simulink model "ConSys_A1"  (Simulink 8.3)
settings: Solver=ode3  StartTime=0.0  StopTime=Time(end)  FixedStep=Ts  RelTol=1e-3
values from neighbouring files (symbols this model uses):
  d = r*h    (= 1.6)    [StartUp_A1.m]
  d0 = d*h    (= 0.0032)    [StartUp_A1.m]
  h = 0.002    [StartUp_A1.m]
  Ka = diag([ 3  20  20  150  355  520])    [StartUp_A1.m]
  Kd = diag([ 3   5  25  100   15 1050])    [StartUp_A1.m]
  Ki = diag([35 555 810 7410 1850 5815])    [StartUp_A1.m]
  Kp = diag([55 180 350 1960  680 4450])    [StartUp_A1.m]
  r = 800    [StartUp_A1.m]
  TD = ss(Atd,Btd,Ctd,Dtd,Ts)    [StartUp_A1.m]
  Ts = 1/200    (= 0.005)    [StartUp_A1.m]
undefined symbols (not defined in the file or in its folder): DiscIntNeverNeededParam
undefined symbols (not defined in the file): ADAMS_cwd, ADAMS_exec, ADAMS_host, ADAMS_init, ADAMS_inputs, ADAMS_outputs, ADAMS_prefix, ADAMS_static, ADAMS_sysdir
libraries: cstblocks x6
(part 5 of 9)

== matlab function A2/MATLAB Function 2 ==
  data: q input double; V2 output double; dq input double
function V2 = V2(q,dq)
%#codegen
Th1=q(1,1); Th2=q(2,1); Th3=q(3,1); Th4=q(4,1); Th5=q(5,1); Th6=q(6,1);
dTh1=dq(1); dTh2=dq(2); dTh3=dq(3); dTh4=dq(4); dTh5=dq(5); dTh6=dq(6);
%---------------------------
V211=(0.34701*cos(Th2) - 0.50841*sin(2.0*Th2) - 0.006265*cos(2.0*Th2 + 2.0*Th3) - 0.04536*cos(2.0*Th2) + 1.3719*sin(2.0*Th2 + 2.0*Th3) - 0.017028*sin(Th2) - 0.096468*cos(Th2)^2 + (0.55399*sin(Th2 + Th3) + 2.34*cos(Th2) + 1.651*cos(Th2)*sin(Th3) + 1.651*cos(Th3)*sin(Th2))*(0.08523*cos(Th2 + Th3) - 0.36*sin(Th2) + 0.254*cos(Th2)*cos(Th3) - 0.254*sin(Th2)*sin(Th3) + 0.07) - 0.5*(cos(Th6)*(sin(Th2 + Th3)*sin(Th5) - 1.0*cos(Th2 + Th3)*cos(Th4)*cos(Th5)) + cos(Th2 + Th3)*sin(Th4)*sin(Th6))*(0.001043*cos(Th6)*(cos(Th2 + Th3)*sin(Th5) + sin(Th2 + Th3)*cos(Th4)*cos(Th5)) - 4.0e-6*cos(Th2 + Th3)*cos(Th5) + 4.0e-6*sin(Th2 + Th3)*cos(Th4)*sin(Th5) - 0.001043*sin(Th2 + Th3)*sin(Th4)*sin(Th6)) - 0.004943*cos(Th2 + Th3)*sin(Th2 + Th3) - 0.5*(sin(Th6)*(cos(Th2 + Th3)*sin(Th5) + sin(Th2 + Th3)*cos(Th4)*cos(Th5)) + sin(Th2 + Th3)*cos(Th6)*sin(Th4))*(0.00104*sin(Th6)*(sin(Th2 + Th3)*sin(Th5) - 1.0*cos(Th2 + Th3)*cos(Th4)*cos(Th5)) - 0.00104*cos(Th2 + Th3)*cos(Th6)*sin(Th4)) - 0.5*(sin(Th6)*(sin(Th2 + Th3)*sin(Th5) - 1.0*cos(Th2 + Th3)*cos(Th4)*cos(Th5)) - 1.0*cos(Th2 + Th3)*cos(Th6)*sin(Th4))*(0.00104*sin(Th6)*(cos(Th2 + Th3)*sin(Th5) + sin(Th2 + Th3)*cos(Th4)*cos(Th5)) + 0.00104*sin(Th2 + Th3)*cos(Th6)*sin(Th4)) + 0.5*(sin(Th2 + Th3)*cos(Th5) + cos(Th2 + Th3)*cos(Th4)*sin(Th5))*(4.0e-6*cos(Th6)*(cos(Th2 + Th3)*sin(Th5) + sin(Th2 + Th3)*cos(Th4)*cos(Th5)) - 0.000116*cos(Th2 + Th3)*cos(Th5) + 0.000116*sin(Th2 + Th3)*cos(Th4)*sin(Th5) - 4.0e-6*sin(Th2 + Th3)*sin(Th4)*sin(Th6)) + 0.5*(cos(Th2 + Th3)*cos(Th5) - 1.0*sin(Th2 + Th3)*cos(Th4)*sin(Th5))*(4.0e-6*cos(Th6)*(sin(Th2 + Th3)*sin(Th5) - 1.0*cos(Th2 + Th3)*cos(Th4)*cos(Th5)) - 0.000116*sin(Th2 + Th3)*cos(Th5) - 0.000116*cos(Th2 + Th3)*cos(Th4)*sin(Th5) + 4.0e-6*cos(Th2 + Th3)*sin(Th4)*sin(Th6)) - 1.0*(0.126*sin(Th2 + Th3) + 0.36*cos(Th2) + 0.00062*cos(Th2 + Th3)*sin(Th4) - 0.00152*sin(Th2 + Th3)*cos(Th5) - 0.00002*sin(Th2 + Th3)*sin(Th5) + 0.254*cos(Th2)*sin(Th3) + 0.254*cos(Th3)*sin(Th2) + 0.00002*cos(Th2 + Th3)*cos(Th4)*cos(Th5) - 0.00152*cos(Th2 + Th3)*cos(Th4)*sin(Th5))*(0.36*sin(Th2) - 0.126*cos(Th2 + Th3) + 0.00152*cos(Th2 + Th3)*cos(Th5) + 0.00002*cos(Th2 + Th3)*sin(Th5) + 0.00062*sin(Th2 + Th3)*sin(Th4) - 0.254*cos(Th2)*cos(Th3) + 0.254*sin(Th2)*sin(Th3) + 0.00002*sin(Th2 + Th3)*cos(Th4)*cos(Th5) - 0.00152*sin(Th2 + Th3)*cos(Th4)*sin(Th5) - 0.07) + (0.063*sin(Th2 + Th3) + 0.18*cos(Th2) + 0.02603*sin(Th2 + Th3)*cos(Th5) + 0.127*cos(Th2)*sin(Th3) + 0.127*cos(Th3)*sin(Th2) + 0.02603*cos(Th2 + Th3)*cos(Th4)*sin(Th5) + 0.000115*cos(Th2 + Th3)*sin(Th4)*sin(Th6) + 0.000115*sin(Th2 + Th3)*cos(Th6)*sin(Th5) - 0.000115*cos(Th2 + Th3)*cos(Th4)*cos(Th5)*cos(Th6))*(0.126*cos(Th2 + Th3) - 0.36*sin(Th2) + 0.05206*cos(Th2 + Th3)*cos(Th5) + 0.254*cos(Th2)*cos(Th3) - 0.254*sin(Th2)*sin(Th3) + 0.00023*cos(Th2 + Th3)*cos(Th6)*sin(Th5) - 0.05206*sin(Th2 + Th3)*cos(Th4)*sin(Th5) - 0.00023*sin(Th2 + Th3)*sin(Th4)*sin(Th6) + 0.00023*sin(Th2 + Th3)*cos(Th4)*cos(Th5)*cos(Th6) + 0.07) + (0.01602*cos(Th2 + Th3) + 2.4568*sin(Th2 + Th3) - 6.48*cos(Th2))*(0.13649*cos(Th2 + Th3) - 0.00089*sin(Th2 + Th3) + 0.36*sin(Th2) - 0.07) - 0.98061*cos(Th2)*sin(Th2) - 0.5*(cos(Th6)*(cos(Th2 + Th3)*sin(Th5) + sin(Th2 + Th3)*cos(Th4)*cos(Th5)) - 1.0*sin(Th2 + Th3)*sin(Th4)*sin(Th6))*(0.001043*cos(Th6)*(sin(Th2 + Th3)*sin(Th5) - 1.0*cos(Th2 + Th3)*cos(Th4)*cos(Th5)) - 4.0e-6*sin(Th2 + Th3)*cos(Th5) - 4.0e-6*cos(Th2 + Th3)*cos(Th4)*sin(Th5) + 0.001043*cos(Th2 + Th3)*sin(Th4)*sin(Th6)) + 0.011125*cos(Th2 + Th3)*sin(Th2 + Th3)*cos(Th4)^2 - 0.000489*cos(Th2 + Th3)*sin(Th2 + Th3)*cos(Th5)^2 + 0.02091*cos(Th2 + Th3)*sin(Th2 + Th3)*sin(Th4)^2 - 0.004898*cos(Th2 + Th3)*sin(Th2 + Th3)*sin(Th5)^2 + 0.00004*cos(Th2 + Th3)^2*cos(Th5)*sin(Th4) - 0.00004*sin(Th2 + Th3)^2*cos(Th5)*sin(Th4) + 0.004409*cos(Th2 + Th3)^2*cos(Th4)*cos(Th5)*sin(Th5) - 0.004409*sin(Th2 + Th3)^2*cos(Th4)*cos(Th5)*sin(Th5) + 0.004898*cos(Th2 + Th3)*sin(Th2 + Th3)*cos(Th4)^2*cos(Th5)^2 + 0.000489*cos(Th2 + Th3)*sin(Th2 + Th3)*cos(Th4)^2*sin(Th5)^2 - 0.00008*cos(Th2 + Th3)*sin(Th2 + Th3)*cos(Th4)*sin(Th4)*sin(Th5) + 0.048234)*dTh1*dTh1;
V212=(0.019809*cos(Th2 + Th3) - 0.000076053*sin(Th2 + Th3) + 0.0008533*cos(Th2) + 0.35821*sin(Th2) - 0.5*(0.00062*cos(Th4) - 0.00002*cos(Th5)*sin(Th4) + 0.00152*sin(Th4)*sin(Th5))*(0.36*sin(Th2) - 0.126*cos(Th2 + Th3) + 0.00152*cos(Th2 + Th3)*cos(Th5) + 0.00002*cos(Th2 + Th3)*sin(Th5) + 0.00062*sin(Th2 + Th3)*sin(Th4) - 0.254*cos(Th2)*cos(Th3) + 0.254*sin(Th2)*sin(Th3) + 0.00002*sin(Th2 + Th3)*cos(Th4)*cos(Th5) - 0.00152*sin(Th2 + Th3)*cos(Th4)*sin(Th5)) + 0.00002*sin(Th2 + Th3)*sin(Th5) + 0.5*(0.000115*cos(Th4)*sin(Th6) - 0.02603*sin(Th4)*sin(Th5) + 0.000115*cos(Th5)*cos(Th6)*sin(Th4))*(0.126*cos(Th2 + Th3) - 0.36*sin(Th2) + 0.05206*cos(Th2 + Th3)*cos(Th5) + 0.254*cos(Th2)*cos(Th3) - 0.254*sin(Th2)*sin(Th3) + 0.00023*cos(Th2 + Th3)*cos(Th6)*sin(Th5) - 0.05206*sin(Th2 + Th3)*cos(Th4)*sin(Th5) - 0.00023*sin(Th2 + Th3)*sin(Th4)*sin(Th6) + 0.00023*sin(Th2 + Th3)*cos(Th4)*cos(Th5)*cos(Th6)) + 0.00002*cos(Th2 + Th3)*cos(Th4)*cos(Th5) - 2.0e-6*cos(Th2 + Th3)*cos(Th6)*sin(Th4) + 0.0051115*sin(Th2 + Th3)*cos(Th4)*sin(Th4) + 2.0e-6*sin(Th2 + Th3)*sin(Th5)*sin(Th6) - 0.00004*sin(Th2 + Th3)*cos(Th4)^2*sin(Th5) + 2.0e-6*cos(Th2 + Th3)*cos(Th4)*cos(Th5)*sin(Th6) - 0.0026665*cos(Th2 + Th3)*cos(Th5)*sin(Th4)*sin(Th5) + 1.5e-6*sin(Th2 + Th3)*cos(Th5)*cos(Th6)*sin(Th6) + 4.0e-6*cos(Th2 + Th3)*cos(Th5)^2*cos(Th6)*sin(Th4) - 0.0026665*sin(Th2 + Th3)*cos(Th4)*cos(Th5)^2*sin(Th4) - 1.5e-6*sin(Th2 + Th3)*cos(Th4)*cos(Th6)^2*sin(Th4) - 4.0e-6*sin(Th2 + Th3)*cos(Th4)^2*sin(Th5)*sin(Th6) - 1.5e-6*cos(Th2 + Th3)*cos(Th5)*cos(Th6)^2*sin(Th4)*sin(Th5) - 3.0e-6*sin(Th2 + Th3)*cos(Th4)^2*cos(Th5)*cos(Th6)*sin(Th6) - 1.5e-6*sin(Th2 + Th3)*cos(Th4)*cos(Th5)^2*cos(Th6)^2*sin(Th4) - 1.5e-6*cos(Th2 + Th3)*cos(Th4)*cos(Th6)*sin(Th5)*sin(Th6) - 4.0e-6*sin(Th2 + Th3)*cos(Th4)*cos(Th5)*cos(Th6)*sin(Th4)*sin(Th5))*dTh1*dTh2;
V213=(0.019809*cos(Th2 + Th3) - 0.000076053*sin(Th2 + Th3) - 0.5*(0.00062*cos(Th4) - 0.00002*cos(Th5)*sin(Th4) + 0.00152*sin(Th4)*sin(Th5))*(0.00152*cos(Th2 + Th3)*cos(Th5) - 0.126*cos(Th2 + Th3) + 0.00002*cos(Th2 + Th3)*sin(Th5) + 0.00062*sin(Th2 + Th3)*sin(Th4) - 0.254*cos(Th2)*cos(Th3) + 0.254*sin(Th2)*sin(Th3) + 0.00002*sin(Th2 + Th3)*cos(Th4)*cos(Th5) - 0.00152*sin(Th2 + Th3)*cos(Th4)*sin(Th5)) + 0.00002*sin(Th2 + Th3)*sin(Th5) + 0.5*(0.000115*cos(Th4)*sin(Th6) - 0.02603*sin(Th4)*sin(Th5) + 0.000115*cos(Th5)*cos(Th6)*sin(Th4))*(0.126*cos(Th2 + Th3) + 0.05206*cos(Th2 + Th3)*cos(Th5) + 0.254*cos(Th2)*cos(Th3) - 0.254*sin(Th2)*sin(Th3) + 0.00023*cos(Th2 + Th3)*cos(Th6)*sin(Th5) - 0.05206*sin(Th2 + Th3)*cos(Th4)*sin(Th5) - 0.00023*sin(Th2 + Th3)*sin(Th4)*sin(Th6) + 0.00023*sin(Th2 + Th3)*cos(Th4)*cos(Th5)*cos(Th6)) + 0.00002*cos(Th2 + Th3)*cos(Th4)*cos(Th5) - 2.0e-6*cos(Th2 + Th3)*cos(Th6)*sin(Th4) + 0.0051115*sin(Th2 + Th3)*cos(Th4)*sin(Th4) + 2.0e-6*sin(Th2 + Th3)*sin(Th5)*sin(Th6) - 0.00004*sin(Th2 + Th3)*cos(Th4)^2*sin(Th5) + 2.0e-6*cos(Th2 + Th3)*cos(Th4)*cos(Th5)*sin(Th6) - 0.0026665*cos(Th2 + Th3)*cos(Th5)*sin(Th4)*sin(Th5) + 1.5e-6*sin(Th2 + Th3)*cos(Th5)*cos(Th6)*sin(Th6) + 4.0e-6*cos(Th2 + Th3)*cos(Th5)^2*cos(Th6)*sin(Th4) - 0.0026665*sin(Th2 + Th3)*cos(Th4)*cos(Th5)^2*sin(Th4) - 1.5e-6*sin(Th2 + Th3)*cos(Th4)*cos(Th6)^2*sin(Th4) - 4.0e-6*sin(Th2 + Th3)*cos(Th4)^2*sin(Th5)*sin(Th6) - 1.5e-6*cos(Th2 + Th3)*cos(Th5)*cos(Th6)^2*sin(Th4)*sin(Th5) - 3.0e-6*sin(Th2 + Th3)*cos(Th4)^2*cos(Th5)*cos(Th6)*sin(Th6) - 1.5e-6*sin(Th2 + Th3)*cos(Th4)*cos(Th5)^2*cos(Th6)^2*sin(Th4) - 1.5e-6*cos(Th2 + Th3)*cos(Th4)*cos(Th6)*sin(Th5)*sin(Th6) - 4.0e-6*sin(Th2 + Th3)*cos(Th4)*cos(Th5)*cos(Th6)*sin(Th4)*sin(Th5))*dTh1*dTh3;
V214=(0.0054606*cos(Th2)*cos(Th3) - 0.0003348*cos(Th2)*sin(Th4) - 0.0054606*sin(Th2)*sin(Th3) + 0.02316*cos(Th4)^2*sin(Th2)*sin(Th3) + 0.0033452*cos(Th5)^2*sin(Th2)*sin(Th3) + 4.4603e-6*cos(Th6)^2*sin(Th2)*sin(Th3) - 0.0000108*cos(Th2)*cos(Th4)*cos(Th5) - 4.56e-8*cos(Th2)*cos(Th4)*sin(Th3) - 4.56e-8*cos(Th3)*cos(Th4)*sin(Th2) - 0.013235*cos(Th2)*cos(Th4)*sin(Th5) - 0.0003534*cos(Th2)*sin(Th3)*sin(Th4) - 0.0003534*cos(Th3)*sin(Th2)*sin(Th4) - 0.0000621*cos(Th2)*sin(Th4)*sin(Th6) - 0.02316*cos(Th2)*cos(Th3)*cos(Th4)^2 - 0.0033452*cos(Th2)*cos(Th3)*cos(Th5)^2 - 4.4603e-6*cos(Th2)*cos(Th3)*cos(Th6)^2 - 0.013381*cos(Th4)^2*cos(Th5)^2*sin(Th2)*sin(Th3) - 5.9471e-6*cos(Th4)^2*cos(Th6)^2*sin(Th2)*sin(Th3) + 1.4868e-6*cos(Th5)^2*cos(Th6)^2*sin(Th2)*sin(Th3) + 0.0000621*cos(Th2)*cos(Th4)*cos(Th5)*cos(Th6) - 0.0000114*cos(Th2)*cos(Th4)*cos(Th5)*sin(Th3) - 0.0000114*cos(Th3)*cos(Th4)*cos(Th5)*sin(Th2) - 3.04e-8*cos(Th2)*cos(Th3)*cos(Th5)*sin(Th5) - 0.00001498*cos(Th2)*cos(Th4)*cos(Th6)*sin(Th3) - 0.00001498*cos(Th3)*cos(Th4)*cos(Th6)*sin(Th2) - 0.013971*cos(Th2)*cos(Th4)*sin(Th3)*sin(Th5) - 0.000058586*cos(Th2)*cos(Th5)*sin(Th3)*sin(Th4) - 0.013971*cos(Th3)*cos(Th4)*sin(Th2)*sin(Th5) - 0.000058586*cos(Th3)*cos(Th5)*sin(Th2)*sin(Th4) + 1.86e-8*cos(Th2)*sin(Th3)*sin(Th4)*sin(Th5) + 1.86e-8*cos(Th3)*sin(Th2)*sin(Th4)*sin(Th5) - 0.00006555*cos(Th2)*sin(Th3)*sin(Th4)*sin(Th6) - 0.00006555*cos(Th3)*sin(Th2)*sin(Th4)*sin(Th6) + 3.04e-8*cos(Th5)*sin(Th2)*sin(Th3)*sin(Th5) + 9.12e-8*cos(Th2)*cos(Th4)*cos(Th5)^2*sin(Th3) + 9.12e-8*cos(Th3)*cos(Th4)*cos(Th5)^2*sin(Th2) + 0.013381*cos(Th2)*cos(Th3)*cos(Th4)^2*cos(Th5)^2 + 5.9471e-6*cos(Th2)*cos(Th3)*cos(Th4)^2*cos(Th6)^2 - 1.4868e-6*cos(Th2)*cos(Th3)*cos(Th5)^2*cos(Th6)^2 - 4.96e-8*cos(Th2)*cos(Th3)*cos(Th4)*cos(Th5)*sin(Th4) + 0.00006555*cos(Th2)*cos(Th4)*cos(Th5)*cos(Th6)*sin(Th3) + 0.00006555*cos(Th3)*cos(Th4)*cos(Th5)*cos(Th6)*sin(Th2) - 9.9869e-6*cos(Th2)*cos(Th3)*cos(Th5)*cos(Th6)*sin(Th5) + 5.9471e-6*cos(Th2)*cos(Th3)*cos(Th4)^2*cos(Th5)^2*cos(Th6)^2 - 0.00015623*cos(Th2)*cos(Th3)*cos(Th4)*sin(Th4)*sin(Th5) - 0.010036*cos(Th2)*cos(Th4)*cos(Th5)*sin(Th3)*sin(Th5) - 0.010036*cos(Th3)*cos(Th4)*cos(Th5)*sin(Th2)*sin(Th5) + 4.96e-8*cos(Th4)*cos(Th5)*sin(Th2)*sin(Th3)*sin(Th4) - 0.00001498*cos(Th2)*cos(Th5)*sin(Th3)*sin(Th4)*sin(Th6) - 0.00001498*cos(Th3)*cos(Th5)*sin(Th2)*sin(Th4)*sin(Th6) + 9.9869e-6*cos(Th5)*cos(Th6)*sin(Th2)*sin(Th3)*sin(Th5) - 5.9471e-6*cos(Th4)^2*cos(Th5)^2*cos(Th6)^2*sin(Th2)*sin(Th3) + 0.00015623*cos(Th4)*sin(Th2)*sin(Th3)*sin(Th4)*sin(Th5) + 1.216e-7*cos(Th2)*cos(Th3)*cos(Th4)^2*cos(Th5)*sin(Th5) + 0.000029961*cos(Th2)*cos(Th4)*cos(Th5)^2*cos(Th6)*sin(Th3) + 0.000029961*cos(Th3)*cos(Th4)*cos(Th5)^2*cos(Th6)*sin(Th2) - 1.216e-7*cos(Th4)^2*cos(Th5)*sin(Th2)*sin(Th3)*sin(Th5) + 0.000039948*cos(Th2)*cos(Th3)*cos(Th4)^2*cos(Th5)*cos(Th6)*sin(Th5) - 4.4603e-6*cos(Th2)*cos(Th4)*cos(Th5)*cos(Th6)^2*sin(Th3)*sin(Th5) - 4.4603e-6*cos(Th3)*cos(Th4)*cos(Th5)*cos(Th6)^2*sin(Th2)*sin(Th5) - 0.000039948*cos(Th4)^2*cos(Th5)*cos(Th6)*sin(Th2)*sin(Th3)*sin(Th5) - 0.000039948*cos(Th2)*cos(Th3)*cos(Th4)*sin(Th4)*sin(Th5)*sin(Th6) + 4.4603e-6*cos(Th2)*cos(Th6)*sin(Th3)*sin(Th4)*sin(Th5)*sin(Th6) + 4.4603e-6*cos(Th3)*cos(Th6)*sin(Th2)*sin(Th4)*sin(Th5)*sin(Th6) + 0.000039948*cos(Th4)*sin(Th2)*sin(Th3)*sin(Th4)*sin(Th5)*sin(Th6) - 0.000011894*cos(Th2)*cos(Th3)*cos(Th4)*cos(Th5)*cos(Th6)*sin(Th4)*sin(Th6) + 0.000011894*cos(Th4)*cos(Th5)*cos(Th6)*sin(Th2)*sin(Th3)*sin(Th4)*sin(Th6))*dTh1*dTh4;
V215=(1.86e-8*cos(Th2)*cos(Th3)*sin(Th5) - 0.000058586*cos(Th2)*cos(Th3)*cos(Th5) - 0.013235*cos(Th2)*cos(Th5)*sin(Th4) + 0.0028942*cos(Th2)*sin(Th3)*sin(Th4) + 0.0028942*cos(Th3)*sin(Th2)*sin(Th4) + 0.000058586*cos(Th5)*sin(Th2)*sin(Th3) + 0.0000108*cos(Th2)*sin(Th4)*sin(Th5) - 1.86e-8*sin(Th2)*sin(Th3)*sin(Th5) - 6.08e-8*cos(Th2)*cos(Th3)*cos(Th4)*sin(Th4) - 6.2e-9*cos(Th2)*cos(Th4)*cos(Th5)*sin(Th3) - 6.2e-9*cos(Th3)*cos(Th4)*cos(Th5)*sin(Th2) - 0.00001498*cos(Th2)*cos(Th3)*cos(Th5)*sin(Th6) - 0.000019529*cos(Th2)*cos(Th4)*sin(Th3)*sin(Th5) - 0.013971*cos(Th2)*cos(Th5)*sin(Th3)*sin(Th4) - 0.000019529*cos(Th3)*cos(Th4)*sin(Th2)*sin(Th5) - 0.013971*cos(Th3)*cos(Th5)*sin(Th2)*sin(Th4) - 0.0000621*cos(Th2)*cos(Th6)*sin(Th4)*sin(Th5) + 6.08e-8*cos(Th4)*sin(Th2)*sin(Th3)*sin(Th4) + 0.0000114*cos(Th2)*sin(Th3)*sin(Th4)*sin(Th5) + 0.0000114*cos(Th3)*sin(Th2)*sin(Th4)*sin(Th5) + 0.00001498*cos(Th5)*sin(Th2)*sin(Th3)*sin(Th6) + 0.000078115*cos(Th2)*cos(Th3)*cos(Th4)^2*cos(Th5) - 2.48e-8*cos(Th2)*cos(Th3)*cos(Th4)^2*sin(Th5) - 0.013381*cos(Th2)*cos(Th5)^2*sin(Th3)*sin(Th4) - 0.013381*cos(Th3)*cos(Th5)^2*sin(Th2)*sin(Th4) - 0.000078115*cos(Th4)^2*cos(Th5)*sin(Th2)*sin(Th3) + 4.4603e-6*cos(Th2)*cos(Th6)^2*sin(Th3)*sin(Th4) + 4.4603e-6*cos(Th3)*cos(Th6)^2*sin(Th2)*sin(Th4) + 2.48e-8*cos(Th4)^2*sin(Th2)*sin(Th3)*sin(Th5) - 0.000019974*cos(Th2)*cos(Th3)*cos(Th4)*cos(Th6)*sin(Th4) + 4.4603e-6*cos(Th2)*cos(Th3)*cos(Th6)*sin(Th5)*sin(Th6) - 1.216e-7*cos(Th2)*cos(Th5)*sin(Th3)*sin(Th4)*sin(Th5) - 1.216e-7*cos(Th3)*cos(Th5)*sin(Th2)*sin(Th4)*sin(Th5) + 0.000019974*cos(Th4)*cos(Th6)*sin(Th2)*sin(Th3)*sin(Th4) - 4.9934e-6*cos(Th2)*cos(Th4)*sin(Th3)*sin(Th5)*sin(Th6) - 0.00006555*cos(Th2)*cos(Th6)*sin(Th3)*sin(Th4)*sin(Th5) - 4.9934e-6*cos(Th3)*cos(Th4)*sin(Th2)*sin(Th5)*sin(Th6) - 0.00006555*cos(Th3)*cos(Th6)*sin(Th2)*sin(Th4)*sin(Th5) - 4.4603e-6*cos(Th6)*sin(Th2)*sin(Th3)*sin(Th5)*sin(Th6) + 1.216e-7*cos(Th2)*cos(Th3)*cos(Th4)*cos(Th5)^2*sin(Th4) + 0.000019974*cos(Th2)*cos(Th3)*cos(Th4)^2*cos(Th5)*sin(Th6) - 1.216e-7*cos(Th4)*cos(Th5)^2*sin(Th2)*sin(Th3)*sin(Th4) - 0.000019974*cos(Th4)^2*cos(Th5)*sin(Th2)*sin(Th3)*sin(Th6) - 5.9471e-6*cos(Th2)*cos(Th5)^2*cos(Th6)^2*sin(Th3)*sin(Th4) - 5.9471e-6*cos(Th3)*cos(Th5)^2*cos(Th6)^2*sin(Th2)*sin(Th4) + 0.000039948*cos(Th2)*cos(Th3)*cos(Th4)*cos(Th5)^2*cos(Th6)*sin(Th4) - 5.9471e-6*cos(Th2)*cos(Th3)*cos(Th4)^2*cos(Th6)*sin(Th5)*sin(Th6) - 0.000039948*cos(Th4)*cos(Th5)^2*cos(Th6)*sin(Th2)*sin(Th3)*sin(Th4) + 5.9471e-6*cos(Th4)^2*cos(Th6)*sin(Th2)*sin(Th3)*sin(Th5)*sin(Th6) - 0.013381*cos(Th2)*cos(Th3)*cos(Th4)*cos(Th5)*sin(Th4)*sin(Th5) - 1.4868e-6*cos(Th2)*cos(Th4)*cos(Th5)*cos(Th6)*sin(Th3)*sin(Th6) - 1.4868e-6*cos(Th3)*cos(Th4)*cos(Th5)*cos(Th6)*sin(Th2)*sin(Th6) - 0.000039948*cos(Th2)*cos(Th5)*cos(Th6)*sin(Th3)*sin(Th4)*sin(Th5) - 0.000039948*cos(Th3)*cos(Th5)*cos(Th6)*sin(Th2)*sin(Th4)*sin(Th5) + 0.013381*cos(Th4)*cos(Th5)*sin(Th2)*sin(Th3)*sin(Th4)*sin(Th5) + 5.9471e-6*cos(Th4)*cos(Th5)*cos(Th6)^2*sin(Th2)*sin(Th3)*sin(Th4)*sin(Th5) - 5.9471e-6*cos(Th2)*cos(Th3)*cos(Th4)*cos(Th5)*cos(Th6)^2*sin(Th4)*sin(Th5))*dTh1*dTh5;
V216=(0.0000621*cos(Th2)*cos(Th4)*cos(Th6) - 0.00005504*cos(Th2)*cos(Th3)*cos(Th5) + 0.00005504*cos(Th5)*sin(Th2)*sin(Th3) + 0.00006555*cos(Th2)*cos(Th4)*cos(Th6)*sin(Th3) + 0.00006555*cos(Th3)*cos(Th4)*cos(Th6)*sin(Th2) - 4.9934e-6*cos(Th2)*cos(Th3)*cos(Th6)*sin(Th5) + 0.000060987*cos(Th2)*cos(Th4)*sin(Th3)*sin(Th5) + 0.000060987*cos(Th3)*cos(Th4)*sin(Th2)*sin(Th5) - 0.0000621*cos(Th2)*cos(Th5)*sin(Th4)*sin(Th6) + 4.9934e-6*cos(Th2)*sin(Th3)*sin(Th4)*sin(Th6) + 4.9934e-6*cos(Th3)*sin(Th2)*sin(Th4)*sin(Th6) + 4.9934e-6*cos(Th6)*sin(Th2)*sin(Th3)*sin(Th5) - 5.9471e-6*cos(Th2)*cos(Th3)*cos(Th4)^2*cos(Th5) - 5.9471e-6*cos(Th2)*cos(Th3)*cos(Th5)*cos(Th6)^2 + 5.9471e-6*cos(Th4)^2*cos(Th5)*sin(Th2)*sin(Th3) + 5.9471e-6*cos(Th5)*cos(Th6)^2*sin(Th2)*sin(Th3) + 0.00001498*cos(Th2)*cos(Th4)*cos(Th5)*cos(Th6)*sin(Th3) + 0.00001498*cos(Th3)*cos(Th4)*cos(Th5)*cos(Th6)*sin(Th2) - 0.00006555*cos(Th2)*cos(Th5)*sin(Th3)*sin(Th4)*sin(Th6) - 0.00006555*cos(Th3)*cos(Th5)*sin(Th2)*sin(Th4)*sin(Th6) + 0.000019974*cos(Th2)*cos(Th3)*cos(Th4)^2*cos(Th6)*sin(Th5) - 5.9471e-6*cos(Th2)*cos(Th4)*cos(Th6)^2*sin(Th3)*sin(Th5) - 5.9471e-6*cos(Th3)*cos(Th4)*cos(Th6)^2*sin(Th2)*sin(Th5) - 0.000019974*cos(Th2)*cos(Th5)^2*sin(Th3)*sin(Th4)*sin(Th6) - 0.000019974*cos(Th3)*cos(Th5)^2*sin(Th2)*sin(Th4)*sin(Th6) - 0.000019974*cos(Th4)^2*cos(Th6)*sin(Th2)*sin(Th3)*sin(Th5) + 0.000011894*cos(Th2)*cos(Th3)*cos(Th4)^2*cos(Th5)*cos(Th6)^2 - 0.000011894*cos(Th4)^2*cos(Th5)*cos(Th6)^2*sin(Th2)*sin(Th3) - 5.9471e-6*cos(Th2)*cos(Th3)*cos(Th4)*cos(Th6)*sin(Th4)*sin(Th6) + 5.9471e-6*cos(Th4)*cos(Th6)*sin(Th2)*sin(Th3)*sin(Th4)*sin(Th6) + 5.9471e-6*cos(Th4)*cos(Th5)^2*cos(Th6)*sin(Th2)*sin(Th3)*sin(Th4)*sin(Th6) - 0.000019974*cos(Th2)*cos(Th3)*cos(Th4)*cos(Th5)*sin(Th4)*sin(Th5)*sin(Th6) + 5.9471e-6*cos(Th2)*cos(Th5)*cos(Th6)*sin(Th3)*sin(Th4)*sin(Th5)*sin(Th6) + 5.9471e-6*cos(Th3)*cos(Th5)*cos(Th6)*sin(Th2)*sin(Th4)*sin(Th5)*sin(Th6) + 0.000019974*cos(Th4)*cos(Th5)*sin(Th2)*sin(Th3)*sin(Th4)*sin(Th5)*sin(Th6) - 5.9471e-6*cos(Th2)*cos(Th3)*cos(Th4)*cos(Th5)^2*cos(Th6)*sin(Th4)*sin(Th6))*dTh1*dTh6;
%---------------------------
V221=(0.000076053*sin(Th2 + Th3) - 0.019809*cos(Th2 + Th3) - 0.0008533*cos(Th2) - 0.35821*sin(Th2) + 0.5*(0.00062*cos(Th4) - 0.00002*cos(Th5)*sin(Th4) + 0.00152*sin(Th4)*sin(Th5))*(0.36*sin(Th2) - 0.126*cos(Th2 + Th3) + 0.00152*cos(Th2 + Th3)*cos(Th5) + 0.00002*cos(Th2 + Th3)*sin(Th5) + 0.00062*sin(Th2 + Th3)*sin(Th4) - 0.254*cos(Th2)*cos(Th3) + 0.254*sin(Th2)*sin(Th3) + 0.00002*sin(Th2 + Th3)*cos(Th4)*cos(Th5) - 0.00152*sin(Th2 + Th3)*cos(Th4)*sin(Th5)) - 0.00002*sin(Th2 + Th3)*sin(Th5) - 0.5*(0.000115*cos(Th4)*sin(Th6) - 0.02603*sin(Th4)*sin(Th5) + 0.000115*cos(Th5)*cos(Th6)*sin(Th4))*(0.126*cos(Th2 + Th3) - 0.36*sin(Th2) + 0.05206*cos(Th2 + Th3)*cos(Th5) + 0.254*cos(Th2)*cos(Th3) - 0.254*sin(Th2)*sin(Th3) + 0.00023*cos(Th2 + Th3)*cos(Th6)*sin(Th5) - 0.05206*sin(Th2 + Th3)*cos(Th4)*sin(Th5) - 0.00023*sin(Th2 + Th3)*sin(Th4)*sin(Th6) + 0.00023*sin(Th2 + Th3)*cos(Th4)*cos(Th5)*cos(Th6)) - 0.00002*cos(Th2 + Th3)*cos(Th4)*cos(Th5) + 2.0e-6*cos(Th2 + Th3)*cos(Th6)*sin(Th4) - 0.0051115*sin(Th2 + Th3)*cos(Th4)*sin(Th4) - 2.0e-6*sin(Th2 + Th3)*sin(Th5)*sin(Th6) + 0.00004*sin(Th2 + Th3)*cos(Th4)^2*sin(Th5) - 2.0e-6*cos(Th2 + Th3)*cos(Th4)*cos(Th5)*sin(Th6) + 0.0026665*cos(Th2 + Th3)*cos(Th5)*sin(Th4)*sin(Th5) - 1.5e-6*sin(Th2 + Th3)*cos(Th5)*cos(Th6)*sin(Th6) - 4.0e-6*cos(Th2 + Th3)*cos(Th5)^2*cos(Th6)*sin(Th4) + 0.0026665*sin(Th2 + Th3)*cos(Th4)*cos(Th5)^2*sin(Th4) + 1.5e-6*sin(Th2 + Th3)*cos(Th4)*cos(Th6)^2*sin(Th4) + 4.0e-6*sin(Th2 + Th3)*cos(Th4)^2*sin(Th5)*sin(Th6) + 1.5e-6*cos(Th2 + Th3)*cos(Th5)*cos(Th6)^2*sin(Th4)*sin(Th5) + 3.0e-6*sin(Th2 + Th3)*cos(Th4)^2*cos(Th5)*cos(Th6)*sin(Th6) + 1.5e-6*sin(Th2 + Th3)*cos(Th4)*cos(Th5)^2*cos(Th6)^2*sin(Th4) + 1.5e-6*cos(Th2 + Th3)*cos(Th4)*cos(Th6)*sin(Th5)*sin(Th6) + 4.0e-6*sin(Th2 + Th3)*cos(Th4)*cos(Th5)*cos(Th6)*sin(Th4)*sin(Th5))*dTh2*dTh1;
V222=(0)*dTh2*dTh2;
V223=(0.22909*cos(Th3) + 0.011534*sin(Th3) + 0.017647*cos(Th3)*cos(Th5) - 0.0000144*cos(Th3)*sin(Th5) - 0.0004464*sin(Th3)*sin(Th4) - 0.0000144*cos(Th4)*cos(Th5)*sin(Th3) + 0.0000828*cos(Th3)*cos(Th6)*sin(Th5) - 0.017647*cos(Th4)*sin(Th3)*sin(Th5) - 0.0000828*sin(Th3)*sin(Th4)*sin(Th6) + 0.0000828*cos(Th4)*cos(Th5)*cos(Th6)*sin(Th3))*dTh2*dTh3;
V224=(4.96e-8*cos(Th4)^2*cos(Th5) - 2.48e-8*cos(Th5) - 0.000078115*sin(Th5) - 0.01158*sin(2.0*Th4) + 0.00015623*cos(Th4)^2*sin(Th5) + 0.0004464*cos(Th3)*cos(Th4) - 0.000019974*sin(Th5)*sin(Th6) + 0.000039948*cos(Th4)^2*sin(Th5)*sin(Th6) - 0.0000144*cos(Th3)*cos(Th5)*sin(Th4) + 0.0000828*cos(Th3)*cos(Th4)*sin(Th6) - 5.9471e-6*cos(Th5)*cos(Th6)*sin(Th6) - 0.017647*cos(Th3)*sin(Th4)*sin(Th5) + 0.013381*cos(Th4)*cos(Th5)^2*sin(Th4) + 5.9471e-6*cos(Th4)*cos(Th6)^2*sin(Th4) + 5.9471e-6*cos(Th4)*cos(Th5)^2*cos(Th6)^2*sin(Th4) + 0.0000828*cos(Th3)*cos(Th5)*cos(Th6)*sin(Th4) + 1.216e-7*cos(Th4)*cos(Th5)*sin(Th4)*sin(Th5) + 0.000011894*cos(Th4)^2*cos(Th5)*cos(Th6)*sin(Th6) + 0.000039948*cos(Th4)*cos(Th5)*cos(Th6)*sin(Th4)*sin(Th5))*dTh2*dTh4;
V225=(6.08e-8*cos(Th4)^2 - 0.0000152*cos(Th5) - 0.000019974*cos(Th6) - 0.018628*sin(Th5) - 0.0066904*sin(2.0*Th5) + 1.216e-7*cos(Th5)^2 + 0.000019974*cos(Th4)^2*cos(Th6) + 0.000039948*cos(Th5)^2*cos(Th6) - 1.216e-7*cos(Th4)^2*cos(Th5)^2 + 0.0000874*cos(Th5)*cos(Th6) - 0.0000144*cos(Th5)*sin(Th3) - 0.017647*sin(Th3)*sin(Th5) - 0.000039948*cos(Th4)^2*cos(Th5)^2*cos(Th6) + 0.017647*cos(Th3)*cos(Th4)*cos(Th5) - 0.0000144*cos(Th3)*cos(Th4)*sin(Th5) + 0.000078115*cos(Th4)*cos(Th5)*sin(Th4) + 0.0000828*cos(Th5)*cos(Th6)*sin(Th3) - 2.48e-8*cos(Th4)*sin(Th4)*sin(Th5) + 0.013381*cos(Th4)^2*cos(Th5)*sin(Th5) - 5.9471e-6*cos(Th5)*cos(Th6)^2*sin(Th5) + 5.9471e-6*cos(Th4)^2*cos(Th5)*cos(Th6)^2*sin(Th5) + 0.0000828*cos(Th3)*cos(Th4)*cos(Th6)*sin(Th5) + 0.000019974*cos(Th4)*cos(Th5)*sin(Th4)*sin(Th6) - 5.9471e-6*cos(Th4)*cos(Th6)*sin(Th4)*sin(Th5)*sin(Th6) - 6.08e-8)*dTh2*dTh5;
V226=(0.0000828*cos(Th3)*cos(Th6)*sin(Th4) - 0.0000874*sin(Th5)*sin(Th6) - 5.9471e-6*cos(Th4)*cos(Th5)*sin(Th4) - 0.000019974*cos(Th5)*sin(Th5)*sin(Th6) - 0.0000828*sin(Th3)*sin(Th5)*sin(Th6) + 5.9471e-6*cos(Th4)^2*cos(Th6)*sin(Th6) - 5.9471e-6*cos(Th5)^2*cos(Th6)*sin(Th6) + 5.9471e-6*cos(Th4)^2*cos(Th5)^2*cos(Th6)*sin(Th6) + 0.0000828*cos(Th3)*cos(Th4)*cos(Th5)*sin(Th6) + 0.000019974*cos(Th4)*cos(Th6)*sin(Th4)*sin(Th5) + 0.000011894*cos(Th4)*cos(Th5)*cos(Th6)^2*sin(Th4) + 0.000019974*cos(Th4)^2*cos(Th5)*sin(Th5)*sin(Th6))*dTh2*dTh6;
%---------------------------
V231=(0.000076053*sin(Th2 + Th3) - 0.019809*cos(Th2 + Th3) + 0.5*(0.00062*cos(Th4) - 0.00002*cos(Th5)*sin(Th4) + 0.00152*sin(Th4)*sin(Th5))*(0.00152*cos(Th2 + Th3)*cos(Th5) - 0.126*cos(Th2 + Th3) + 0.00002*cos(Th2 + Th3)*sin(Th5) + 0.00062*sin(Th2 + Th3)*sin(Th4) - 0.254*cos(Th2)*cos(Th3) + 0.254*sin(Th2)*sin(Th3) + 0.00002*sin(Th2 + Th3)*cos(Th4)*cos(Th5) - 0.00152*sin(Th2 + Th3)*cos(Th4)*sin(Th5)) - 0.00002*sin(Th2 + Th3)*sin(Th5) - 0.5*(0.000115*cos(Th4)*sin(Th6) - 0.02603*sin(Th4)*sin(Th5) + 0.000115*cos(Th5)*cos(Th6)*sin(Th4))*(0.126*cos(Th2 + Th3) + 0.05206*cos(Th2 + Th3)*cos(Th5) + 0.254*cos(Th2)*cos(Th3) - 0.254*sin(Th2)*sin(Th3) + 0.00023*cos(Th2 + Th3)*cos(Th6)*sin(Th5) - 0.05206*sin(Th2 + Th3)*cos(Th4)*sin(Th5) - 0.00023*sin(Th2 + Th3)*sin(Th4)*sin(Th6) + 0.00023*sin(Th2 + Th3)*cos(Th4)*cos(Th5)*cos(Th6)) - 0.00002*cos(Th2 + Th3)*cos(Th4)*cos(Th5) + 2.0e-6*cos(Th2 + Th3)*cos(Th6)*sin(Th4) - 0.0051115*sin(Th2 + Th3)*cos(Th4)*sin(Th4) - 2.0e-6*sin(Th2 + Th3)*sin(Th5)*sin(Th6) + 0.00004*sin(Th2 + Th3)*cos(Th4)^2*sin(Th5) - 2.0e-6*cos(Th2 + Th3)*cos(Th4)*cos(Th5)*sin(Th6) + 0.0026665*cos(Th2 + Th3)*cos(Th5)*sin(Th4)*sin(Th5) - 1.5e-6*sin(Th2 + Th3)*cos(Th5)*cos(Th6)*sin(Th6) - 4.0e-6*cos(Th2 + Th3)*cos(Th5)^2*cos(Th6)*sin(Th4) + 0.0026665*sin(Th2 + Th3)*cos(Th4)*cos(Th5)^2*sin(Th4) + 1.5e-6*sin(Th2 + Th3)*cos(Th4)*cos(Th6)^2*sin(Th4) + 4.0e-6*sin(Th2 + Th3)*cos(Th4)^2*sin(Th5)*sin(Th6) + 1.5e-6*cos(Th2 + Th3)*cos(Th5)*cos(Th6)^2*sin(Th4)*sin(Th5) + 3.0e-6*sin(Th2 + Th3)*cos(Th4)^2*cos(Th5)*cos(Th6)*sin(Th6) + 1.5e-6*sin(Th2 + Th3)*cos(Th4)*cos(Th5)^2*cos(Th6)^2*sin(Th4) + 1.5e-6*cos(Th2 + Th3)*cos(Th4)*cos(Th6)*sin(Th5)*sin(Th6) + 4.0e-6*sin(Th2 + Th3)*cos(Th4)*cos(Th5)*cos(Th6)*sin(Th4)*sin(Th5))*dTh3*dTh1;
V232=(0)*dTh3*dTh2;
V233=(0.11454*cos(Th3) + 0.0057672*sin(Th3) + 0.0088236*cos(Th3)*cos(Th5) - 7.2e-6*cos(Th3)*sin(Th5) - 0.0002232*sin(Th3)*sin(Th4) - 7.2e-6*cos(Th4)*cos(Th5)*sin(Th3) + 0.0000414*cos(Th3)*cos(Th6)*sin(Th5) - 0.0088236*cos(Th4)*sin(Th3)*sin(Th5) - 0.0000414*sin(Th3)*sin(Th4)*sin(Th6) + 0.0000414*cos(Th4)*cos(Th5)*cos(Th6)*sin(Th3))*dTh3*dTh3;
V234=(4.96e-8*cos(Th4)^2*cos(Th5) - 2.48e-8*cos(Th5) - 0.000078115*sin(Th5) - 0.01158*sin(2.0*Th4) + 0.00015623*cos(Th4)^2*sin(Th5) + 0.0002232*cos(Th3)*cos(Th4) - 0.000019974*sin(Th5)*sin(Th6) + 0.000039948*cos(Th4)^2*sin(Th5)*sin(Th6) - 7.2e-6*cos(Th3)*cos(Th5)*sin(Th4) + 0.0000414*cos(Th3)*cos(Th4)*sin(Th6) - 5.9471e-6*cos(Th5)*cos(Th6)*sin(Th6) - 0.0088236*cos(Th3)*sin(Th4)*sin(Th5) + 0.013381*cos(Th4)*cos(Th5)^2*sin(Th4) + 5.9471e-6*cos(Th4)*cos(Th6)^2*sin(Th4) + 5.9471e-6*cos(Th4)*cos(Th5)^2*cos(Th6)^2*sin(Th4) + 0.0000414*cos(Th3)*cos(Th5)*cos(Th6)*sin(Th4) + 1.216e-7*cos(Th4)*cos(Th5)*sin(Th4)*sin(Th5) + 0.000011894*cos(Th4)^2*cos(Th5)*cos(Th6)*sin(Th6) + 0.000039948*cos(Th4)*cos(Th5)*cos(Th6)*sin(Th4)*sin(Th5))*dTh3*dTh4;
V235=(6.08e-8*cos(Th4)^2 - 0.0000152*cos(Th5) - 0.000019974*cos(Th6) - 0.018628*sin(Th5) - 0.0066904*sin(2.0*Th5) + 1.216e-7*cos(Th5)^2 + 0.000019974*cos(Th4)^2*cos(Th6) + 0.000039948*cos(Th5)^2*cos(Th6) - 1.216e-7*cos(Th4)^2*cos(Th5)^2 + 0.0000874*cos(Th5)*cos(Th6) - 7.2e-6*cos(Th5)*sin(Th3) - 0.0088236*sin(Th3)*sin(Th5) - 0.000039948*cos(Th4)^2*cos(Th5)^2*cos(Th6) + 0.0088236*cos(Th3)*cos(Th4)*cos(Th5) - 7.2e-6*cos(Th3)*cos(Th4)*sin(Th5) + 0.000078115*cos(Th4)*cos(Th5)*sin(Th4) + 0.0000414*cos(Th5)*cos(Th6)*sin(Th3) - 2.48e-8*cos(Th4)*sin(Th4)*sin(Th5) + 0.013381*cos(Th4)^2*cos(Th5)*sin(Th5) - 5.9471e-6*cos(Th5)*cos(Th6)^2*sin(Th5) + 5.9471e-6*cos(Th4)^2*cos(Th5)*cos(Th6)^2*sin(Th5) + 0.0000414*cos(Th3)*cos(Th4)*cos(Th6)*sin(Th5) + 0.000019974*cos(Th4)*cos(Th5)*sin(Th4)*sin(Th6) - 5.9471e-6*cos(Th4)*cos(Th6)*sin(Th4)*sin(Th5)*sin(Th6) - 6.08e-8)*dTh3*dTh5;
V236=(0.0000414*cos(Th3)*cos(Th6)*sin(Th4) - 0.0000874*sin(Th5)*sin(Th6) - 5.9471e-6*cos(Th4)*cos(Th5)*sin(Th4) - 0.000019974*cos(Th5)*sin(Th5)*sin(Th6) - 0.0000414*sin(Th3)*sin(Th5)*sin(Th6) + 5.9471e-6*cos(Th4)^2*cos(Th6)*sin(Th6) - 5.9471e-6*cos(Th5)^2*cos(Th6)*sin(Th6) + 5.9471e-6*cos(Th4)^2*cos(Th5)^2*cos(Th6)*sin(Th6) + 0.0000414*cos(Th3)*cos(Th4)*cos(Th5)*sin(Th6) + 0.000019974*cos(Th4)*cos(Th6)*sin(Th4)*sin(Th5) + 0.000011894*cos(Th4)*cos(Th5)*cos(Th6)^2*sin(Th4) + 0.000019974*cos(Th4)^2*cos(Th5)*sin(Th5)*sin(Th6))*dTh3*dTh6;
%---------------------------
V241=(0.0061194*sin(Th2)*sin(Th3) - 0.0001116*cos(Th2)*sin(Th4) - 0.0061194*cos(Th2)*cos(Th3) - 0.0033452*cos(Th5)^2*sin(Th2)*sin(Th3) + 1.4868e-6*cos(Th6)^2*sin(Th2)*sin(Th3) - 3.6e-6*cos(Th2)*cos(Th4)*cos(Th5) - 1.52e-8*cos(Th2)*cos(Th4)*sin(Th3) - 1.52e-8*cos(Th3)*cos(Th4)*sin(Th2) - 0.0044118*cos(Th2)*cos(Th4)*sin(Th5) - 0.0001178*cos(Th2)*sin(Th3)*sin(Th4) - 0.0001178*cos(Th3)*sin(Th2)*sin(Th4) - 0.0000207*cos(Th2)*sin(Th4)*sin(Th6) + 0.0033452*cos(Th2)*cos(Th3)*cos(Th5)^2 - 1.4868e-6*cos(Th2)*cos(Th3)*cos(Th6)^2 - 1.4868e-6*cos(Th5)^2*cos(Th6)^2*sin(Th2)*sin(Th3) + 0.0000207*cos(Th2)*cos(Th4)*cos(Th5)*cos(Th6) - 3.8e-6*cos(Th2)*cos(Th4)*cos(Th5)*sin(Th3) - 3.8e-6*cos(Th3)*cos(Th4)*cos(Th5)*sin(Th2) + 3.04e-8*cos(Th2)*cos(Th3)*cos(Th5)*sin(Th5) - 4.9934e-6*cos(Th2)*cos(Th4)*cos(Th6)*sin(Th3) - 4.9934e-6*cos(Th3)*cos(Th4)*cos(Th6)*sin(Th2) - 0.0046569*cos(Th2)*cos(Th4)*sin(Th3)*sin(Th5) - 0.000019529*cos(Th2)*cos(Th5)*sin(Th3)*sin(Th4) - 0.0046569*cos(Th3)*cos(Th4)*sin(Th2)*sin(Th5) - 0.000019529*cos(Th3)*cos(Th5)*sin(Th2)*sin(Th4) + 6.2e-9*cos(Th2)*sin(Th3)*sin(Th4)*sin(Th5) + 6.2e-9*cos(Th3)*sin(Th2)*sin(Th4)*sin(Th5) - 0.00002185*cos(Th2)*sin(Th3)*sin(Th4)*sin(Th6) - 0.00002185*cos(Th3)*sin(Th2)*sin(Th4)*sin(Th6) - 3.04e-8*cos(Th5)*sin(Th2)*sin(Th3)*sin(Th5) + 3.04e-8*cos(Th2)*cos(Th4)*cos(Th5)^2*sin(Th3) + 3.04e-8*cos(Th3)*cos(Th4)*cos(Th5)^2*sin(Th2) + 1.4868e-6*cos(Th2)*cos(Th3)*cos(Th5)^2*cos(Th6)^2 + 0.00002185*cos(Th2)*cos(Th4)*cos(Th5)*cos(Th6)*sin(Th3) + 0.00002185*cos(Th3)*cos(Th4)*cos(Th5)*cos(Th6)*sin(Th2) + 9.9869e-6*cos(Th2)*cos(Th3)*cos(Th5)*cos(Th6)*sin(Th5) - 0.0033452*cos(Th2)*cos(Th4)*cos(Th5)*sin(Th3)*sin(Th5) - 0.0033452*cos(Th3)*cos(Th4)*cos(Th5)*sin(Th2)*sin(Th5) - 4.9934e-6*cos(Th2)*cos(Th5)*sin(Th3)*sin(Th4)*sin(Th6) - 4.9934e-6*cos(Th3)*cos(Th5)*sin(Th2)*sin(Th4)*sin(Th6) - 9.9869e-6*cos(Th5)*cos(Th6)*sin(Th2)*sin(Th3)*sin(Th5) + 9.9869e-6*cos(Th2)*cos(Th4)*cos(Th5)^2*cos(Th6)*sin(Th3) + 9.9869e-6*cos(Th3)*cos(Th4)*cos(Th5)^2*cos(Th6)*sin(Th2) - 1.4868e-6*cos(Th2)*cos(Th4)*cos(Th5)*cos(Th6)^2*sin(Th3)*sin(Th5) - 1.4868e-6*cos(Th3)*cos(Th4)*cos(Th5)*cos(Th6)^2*sin(Th2)*sin(Th5) + 1.4868e-6*cos(Th2)*cos(Th6)*sin(Th3)*sin(Th4)*sin(Th5)*sin(Th6) + 1.4868e-6*cos(Th3)*cos(Th6)*sin(Th2)*sin(Th4)*sin(Th5)*sin(Th6))*dTh4*dTh1;
V242=(0)*dTh4*dTh2;
V243=(1.8e-6*cos(Th3)*(124.0*cos(Th4) - 4.0*cos(Th5)*sin(Th4) + 23.0*cos(Th4)*sin(Th6) - 4902.0*sin(Th4)*sin(Th5) + 23.0*cos(Th5)*cos(Th6)*sin(Th4)))*dTh4*dTh3;
V244=(6.08e-8*cos(Th4)*cos(Th5)^2 - 0.0002356*sin(Th4) - 3.04e-8*cos(Th4) - 7.6e-6*cos(Th4)*cos(Th5) - 9.9869e-6*cos(Th4)*cos(Th6) - 0.0093138*cos(Th4)*sin(Th5) - 0.000039058*cos(Th5)*sin(Th4) - 0.0002232*sin(Th3)*sin(Th4) + 1.24e-8*sin(Th4)*sin(Th5) - 0.0000437*sin(Th4)*sin(Th6) + 0.0000437*cos(Th4)*cos(Th5)*cos(Th6) - 7.2e-6*cos(Th4)*cos(Th5)*sin(Th3) - 0.0066904*cos(Th4)*cos(Th5)*sin(Th5) - 0.0088236*cos(Th4)*sin(Th3)*sin(Th5) - 9.9869e-6*cos(Th5)*sin(Th4)*sin(Th6) - 0.0000414*sin(Th3)*sin(Th4)*sin(Th6) + 0.000019974*cos(Th4)*cos(Th5)^2*cos(Th6) + 0.0000414*cos(Th4)*cos(Th5)*cos(Th6)*sin(Th3) + 2.9736e-6*cos(Th6)*sin(Th4)*sin(Th5)*sin(Th6) - 2.9736e-6*cos(Th4)*cos(Th5)*cos(Th6)^2*sin(Th5))*dTh4*dTh4;
V245=(0.0066904*sin(Th4) - 0.013381*cos(Th5)^2*sin(Th4) + 2.9736e-6*cos(Th6)^2*sin(Th4) - 1.24e-8*cos(Th4)*cos(Th5) - 0.000039058*cos(Th4)*sin(Th5) - 0.0093138*cos(Th5)*sin(Th4) + 7.6e-6*sin(Th4)*sin(Th5) - 5.9471e-6*cos(Th5)^2*cos(Th6)^2*sin(Th4) - 0.0088236*cos(Th5)*sin(Th3)*sin(Th4) - 1.216e-7*cos(Th5)*sin(Th4)*sin(Th5) - 9.9869e-6*cos(Th4)*sin(Th5)*sin(Th6) - 0.0000437*cos(Th6)*sin(Th4)*sin(Th5) + 7.2e-6*sin(Th3)*sin(Th4)*sin(Th5) - 2.9736e-6*cos(Th4)*cos(Th5)*cos(Th6)*sin(Th6) - 0.000039948*cos(Th5)*cos(Th6)*sin(Th4)*sin(Th5) - 0.0000414*cos(Th6)*sin(Th3)*sin(Th4)*sin(Th5))*dTh4*dTh5;
V246=(0.0000437*cos(Th4)*cos(Th6) + 2.9736e-6*cos(Th4)*sin(Th5) + 9.9869e-6*sin(Th4)*sin(Th6) - 0.000019974*cos(Th5)^2*sin(Th4)*sin(Th6) + 9.9869e-6*cos(Th4)*cos(Th5)*cos(Th6) + 0.0000414*cos(Th4)*cos(Th6)*sin(Th3) - 0.0000437*cos(Th5)*sin(Th4)*sin(Th6) - 5.9471e-6*cos(Th4)*cos(Th6)^2*sin(Th5) - 0.0000414*cos(Th5)*sin(Th3)*sin(Th4)*sin(Th6) + 5.9471e-6*cos(Th5)*cos(Th6)*sin(Th4)*sin(Th5)*sin(Th6))*dTh4*dTh6;
%---------------------------
V251=(6.2e-9*cos(Th2)*cos(Th3)*sin(Th5) - 0.000019529*cos(Th2)*cos(Th3)*cos(Th5) - 0.0044118*cos(Th2)*cos(Th5)*sin(Th4) - 0.0037962*cos(Th2)*sin(Th3)*sin(Th4) - 0.0037962*cos(Th3)*sin(Th2)*sin(Th4) + 0.000019529*cos(Th5)*sin(Th2)*sin(Th3) + 3.6e-6*cos(Th2)*sin(Th4)*sin(Th5) - 6.2e-9*sin(Th2)*sin(Th3)*sin(Th5) + 6.2e-9*cos(Th2)*cos(Th4)*cos(Th5)*sin(Th3) + 6.2e-9*cos(Th3)*cos(Th4)*cos(Th5)*sin(Th2) - 4.9934e-6*cos(Th2)*cos(Th3)*cos(Th5)*sin(Th6) + 0.000019529*cos(Th2)*cos(Th4)*sin(Th3)*sin(Th5) - 0.0046569*cos(Th2)*cos(Th5)*sin(Th3)*sin(Th4) + 0.000019529*cos(Th3)*cos(Th4)*sin(Th2)*sin(Th5) - 0.0046569*cos(Th3)*cos(Th5)*sin(Th2)*sin(Th4) - 0.0000207*cos(Th2)*cos(Th6)*sin(Th4)*sin(Th5) + 3.8e-6*cos(Th2)*sin(Th3)*sin(Th4)*sin(Th5) + 3.8e-6*cos(Th3)*sin(Th2)*sin(Th4)*sin(Th5) + 4.9934e-6*cos(Th5)*sin(Th2)*sin(Th3)*sin(Th6) + 1.4868e-6*cos(Th2)*cos(Th6)^2*sin(Th3)*sin(Th4) + 1.4868e-6*cos(Th3)*cos(Th6)^2*sin(Th2)*sin(Th4) + 1.4868e-6*cos(Th2)*cos(Th3)*cos(Th6)*sin(Th5)*sin(Th6) + 4.9934e-6*cos(Th2)*cos(Th4)*sin(Th3)*sin(Th5)*sin(Th6) - 0.00002185*cos(Th2)*cos(Th6)*sin(Th3)*sin(Th4)*sin(Th5) + 4.9934e-6*cos(Th3)*cos(Th4)*sin(Th2)*sin(Th5)*sin(Th6) - 0.00002185*cos(Th3)*cos(Th6)*sin(Th2)*sin(Th4)*sin(Th5) - 1.4868e-6*cos(Th6)*sin(Th2)*sin(Th3)*sin(Th5)*sin(Th6) + 1.4868e-6*cos(Th2)*cos(Th4)*cos(Th5)*cos(Th6)*sin(Th3)*sin(Th6) + 1.4868e-6*cos(Th3)*cos(Th4)*cos(Th5)*cos(Th6)*sin(Th2)*sin(Th6))*dTh5*dTh1;
V252=(0)*dTh5*dTh2;
V253=(0.0088236*cos(Th3)*cos(Th4)*cos(Th5) - 0.0088236*sin(Th3)*sin(Th5) - 7.2e-6*cos(Th5)*sin(Th3) - 7.2e-6*cos(Th3)*cos(Th4)*sin(Th5) + 0.0000414*cos(Th5)*cos(Th6)*sin(Th3) + 0.0000414*cos(Th3)*cos(Th4)*cos(Th6)*sin(Th5))*dTh5*dTh3;
V254=(2.9736e-6*cos(Th6)^2*sin(Th4) - 0.0075924*sin(Th4) + 1.24e-8*cos(Th4)*cos(Th5) + 0.000039058*cos(Th4)*sin(Th5) - 0.0093138*cos(Th5)*sin(Th4) + 7.6e-6*sin(Th4)*sin(Th5) - 0.0088236*cos(Th5)*sin(Th3)*sin(Th4) + 9.9869e-6*cos(Th4)*sin(Th5)*sin(Th6) - 0.0000437*cos(Th6)*sin(Th4)*sin(Th5) + 7.2e-6*sin(Th3)*sin(Th4)*sin(Th5) + 2.9736e-6*cos(Th4)*cos(Th5)*cos(Th6)*sin(Th6) - 0.0000414*cos(Th6)*sin(Th3)*sin(Th4)*sin(Th5))*dTh5*dTh4;
V255=(0.0088236*cos(Th3)*cos(Th5) - 7.6e-6*cos(Th4)*cos(Th5) - 7.2e-6*cos(Th3)*sin(Th5) - 0.0093138*cos(Th4)*sin(Th5) + 0.000039058*cos(Th5)*sin(Th4) - 1.24e-8*sin(Th4)*sin(Th5) + 0.0000437*cos(Th4)*cos(Th5)*cos(Th6) - 7.2e-6*cos(Th4)*cos(Th5)*sin(Th3) + 0.0000414*cos(Th3)*cos(Th6)*sin(Th5) - 0.0088236*cos(Th4)*sin(Th3)*sin(Th5) + 9.9869e-6*cos(Th5)*sin(Th4)*sin(Th6) + 0.0000414*cos(Th4)*cos(Th5)*cos(Th6)*sin(Th3) - 2.9736e-6*cos(Th6)*sin(Th4)*sin(Th5)*sin(Th6))*dTh5*dTh5;
V256=(0.0000414*cos(Th3)*cos(Th5)*sin(Th6) - 2.9736e-6*cos(Th5)*sin(Th4) + 5.9471e-6*cos(Th4)*cos(Th6)*sin(Th6) - 0.0000437*cos(Th4)*sin(Th5)*sin(Th6) + 9.9869e-6*cos(Th6)*sin(Th4)*sin(Th5) + 5.9471e-6*cos(Th5)*cos(Th6)^2*sin(Th4) - 0.0000414*cos(Th4)*sin(Th3)*sin(Th5)*sin(Th6))*dTh5*dTh6;
%---------------------------
V261=(0.0000207*cos(Th2)*cos(Th4)*cos(Th6) - 0.000058013*cos(Th2)*cos(Th3)*cos(Th5) + 0.000058013*cos(Th5)*sin(Th2)*sin(Th3) + 0.00002185*cos(Th2)*cos(Th4)*cos(Th6)*sin(Th3) + 0.00002185*cos(Th3)*cos(Th4)*cos(Th6)*sin(Th2) + 4.9934e-6*cos(Th2)*cos(Th3)*cos(Th6)*sin(Th5) + 0.000058013*cos(Th2)*cos(Th4)*sin(Th3)*sin(Th5) + 0.000058013*cos(Th3)*cos(Th4)*sin(Th2)*sin(Th5) - 0.0000207*cos(Th2)*cos(Th5)*sin(Th4)*sin(Th6) - 4.9934e-6*cos(Th2)*sin(Th3)*sin(Th4)*sin(Th6) - 4.9934e-6*cos(Th3)*sin(Th2)*sin(Th4)*sin(Th6) - 4.9934e-6*cos(Th6)*sin(Th2)*sin(Th3)*sin(Th5) + 4.9934e-6*cos(Th2)*cos(Th4)*cos(Th5)*cos(Th6)*sin(Th3) + 4.9934e-6*cos(Th3)*cos(Th4)*cos(Th5)*cos(Th6)*sin(Th2) - 0.00002185*cos(Th2)*cos(Th5)*sin(Th3)*sin(Th4)*sin(Th6) - 0.00002185*cos(Th3)*cos(Th5)*sin(Th2)*sin(Th4)*sin(Th6))*dTh6*dTh1;
V262=(0)*dTh6*dTh2;
V263=(0.0000414*cos(Th3)*cos(Th6)*sin(Th4) - 0.0000414*sin(Th3)*sin(Th5)*sin(Th6) + 0.0000414*cos(Th3)*cos(Th4)*cos(Th5)*sin(Th6))*dTh6*dTh3;
V264=(0.0000437*cos(Th4)*cos(Th6) + 0.00011603*cos(Th4)*sin(Th5) - 9.9869e-6*sin(Th4)*sin(Th6) + 9.9869e-6*cos(Th4)*cos(Th5)*cos(Th6) + 0.0000414*cos(Th4)*cos(Th6)*sin(Th3) - 0.0000437*cos(Th5)*sin(Th4)*sin(Th6) - 0.0000414*cos(Th5)*sin(Th3)*sin(Th4)*sin(Th6))*dTh6*dTh4;
V265=(0.00011603*cos(Th5)*sin(Th4) + 0.0000414*cos(Th3)*cos(Th5)*sin(Th6) - 0.0000437*cos(Th4)*sin(Th5)*sin(Th6) - 9.9869e-6*cos(Th6)*sin(Th4)*sin(Th5) - 0.0000414*cos(Th4)*sin(Th3)*sin(Th5)*sin(Th6))*dTh6*dTh5;
V266=(9.9869e-6*cos(Th4)*cos(Th6) - 0.0000437*sin(Th4)*sin(Th6) + 0.0000437*cos(Th4)*cos(Th5)*cos(Th6) + 0.0000414*cos(Th3)*cos(Th6)*sin(Th5) - 9.9869e-6*cos(Th5)*sin(Th4)*sin(Th6) - 0.0000414*sin(Th3)*sin(Th4)*sin(Th6) + 0.0000414*cos(Th4)*cos(Th5)*cos(Th6)*sin(Th3))*dTh6*dTh6;
%---------------------------
V2 = V211+V212+V213+V214+V215+V216+V221+V222+V223+V224+V225+V226+...
     V231+V232+V233+V234+V235+V236+V241+V242+V243+V244+V245+V246+...
     V251+V252+V253+V254+V255+V256+V261+V262+V263+V264+V265+V266;
end
